simulink model "pendulo_simples"  (R2013a)
settings: Solver=ode3  StartTime=0.0  StopTime=10.0  FixedStep=0.01  RelTol=1e-3
values from neighbouring files (symbols this model uses):
  a =     [lab7.mat]
  b =     [lab7.mat]
undefined symbols (not defined in the file or in its folder): x_1_0, x_2_0
settings Model: Creator=09884147914  LastModifiedBy=09884147914

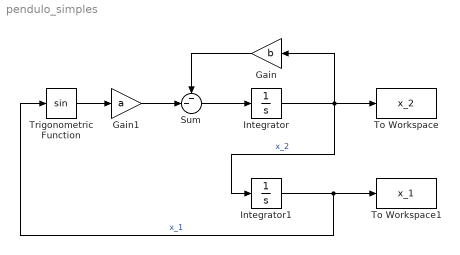
== system pendulo_simples ==
  Gain : Gain  Gain=b
  Gain1 : Gain  Gain=a
  Integrator : Integrator  InitialCondition=x_2_0
  Integrator1 : Integrator  InitialCondition=x_1_0
  Sum : Sum  Inputs=--|
  To Workspace : ToWorkspace  VariableName=x_2  SampleTime=-1  SaveFormat=Timeseries
  To Workspace1 : ToWorkspace  VariableName=x_1  SampleTime=-1  SaveFormat=Timeseries
  Trigonometric Function : Trigonometry
  wires:
  Integrator/1 -> To Workspace/1, Integrator1/1, Gain/1  "x_2"
  Integrator1/1 -> To Workspace1/1, Trigonometric Function/1  "x_1"
  Trigonometric Function/1 -> Gain1/1
  Gain/1 -> Sum/1
  Gain1/1 -> Sum/2
  Sum/1 -> Integrator/1
